simulink model "lab_1"  (R2025a)
settings: Solver=VariableStepAuto  StartTime=0.0  StopTime=20  RelTol=1e-3
model workspace (MAT data in the model file):
  K = Simulink.Parameter
  K.Value = 1.2
  K.Complexity = 'real'
  K.Dimensions = [1 1]
  K.DataType = 'auto'
  N = Simulink.Parameter
  N.Value = 100
  N.Complexity = 'real'
  N.Dimensions = [1 1]
  N.DataType = 'auto'
  T = Simulink.Parameter
  T.Value = 2.1
  T.Complexity = 'real'
  T.Dimensions = [1 1]
  T.DataType = 'auto'
  T_1 = Simulink.Parameter
  T_1.Value = 3.3
  T_1.Complexity = 'real'
  T_1.Dimensions = [1 1]
  T_1.DataType = 'auto'
  T_2 = Simulink.Parameter
  T_2.Value = 1.5
  T_2.Complexity = 'real'
  T_2.Dimensions = [1 1]
  T_2.DataType = 'auto'
  c_1 = Simulink.Parameter
  c_1.Value = 0.1
  c_1.Complexity = 'real'
  c_1.Dimensions = [1 1]
  c_1.DataType = 'auto'
  c_2 = Simulink.Parameter
  c_2.Value = 0.3
  c_2.Complexity = 'real'
  c_2.Dimensions = [1 1]
  c_2.DataType = 'auto'
  c_3 = Simulink.Parameter
  c_3.Value = 0.5
  c_3.Complexity = 'real'
  c_3.Dimensions = [1 1]
  c_3.DataType = 'auto'
settings Model: Creator=konstantin  LastModifiedBy=konstantin

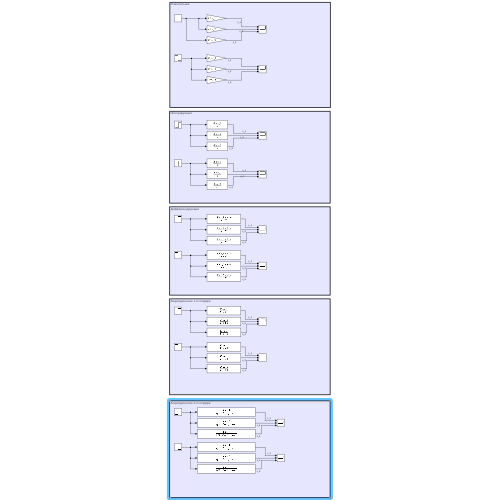
[thumbnail: Simulink's stored preview of the top-level diagram]
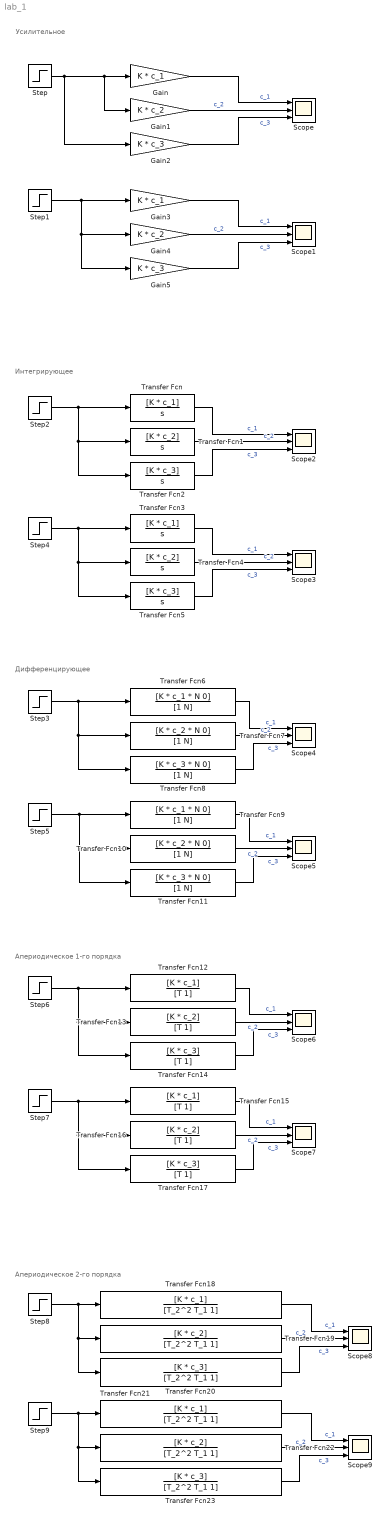
== system lab_1 ==
  note: Апериодическое 2-го порядка
  note: Апериодическое 1-го порядка
  note: Дифференцирующее
  note: Интегрирующее
  note: Усилительное
  Gain : Gain  Gain=K * c_1
  Gain1 : Gain  Gain=K * c_2
  Gain2 : Gain  Gain=K * c_3
  Gain3 : Gain  Gain=K * c_1
  Gain4 : Gain  Gain=K * c_2
  Gain5 : Gain  Gain=K * c_3
  Scope{,1..9} (10 alike) : Scope  NumInputPorts=3
      Scope settings: ActiveDisplayYMinimum=-1  ActiveDisplayYMaximum=1
      Scope1 settings: ActiveDisplayYMinimum=27.339308979558851  ActiveDisplayYMaximum=40.428766776937692
      Scope2 settings: ActiveDisplayYMinimum=-0.74999999999999978  ActiveDisplayYMaximum=6.75  DataLoggingVariableName=ScopeData2
      Scope3 settings: ActiveDisplayYMinimum=-0.74999999999999978  ActiveDisplayYMaximum=6.75  DataLoggingVariableName=ScopeData3
      Scope4 settings: ActiveDisplayYMinimum=-7.4999999999999982  ActiveDisplayYMaximum=67.5  DataLoggingVariableName=ScopeData4
      Scope5 settings: ActiveDisplayYMinimum=-7.4999999999999982  ActiveDisplayYMaximum=67.5  DataLoggingVariableName=ScopeData5
      Scope6 settings: ActiveDisplayYMinimum=-0.073967715995019639  ActiveDisplayYMaximum=0.66570944395517684  DataLoggingVariableName=ScopeData6
      Scope7 settings: ActiveDisplayYMinimum=-0.073967715995019639  ActiveDisplayYMaximum=0.66570944395517684  DataLoggingVariableName=ScopeData7
      Scope8 settings: ActiveDisplayYMinimum=-0.074962390858454561  ActiveDisplayYMaximum=0.67466151772609118  DataLoggingVariableName=ScopeData8
      Scope9 settings: ActiveDisplayYMinimum=-0.01724047204888899  ActiveDisplayYMaximum=0.15516424844000093  DataLoggingVariableName=ScopeData9
  Step : Step  Time=0  SampleTime=0
  Step{1,4..5,7,9} (5 alike) : Step  Time=0.01  Before=100  After=0  SampleTime=0
  Step2 : Step  Time=0  SampleTime=0
  Step3 : Step  SampleTime=0
  Step6 : Step  SampleTime=0
  Step8 : Step  SampleTime=0
  Transfer Fcn : TransferFcn  Numerator=[K * c_1]  Denominator=[1 0]
  Transfer Fcn1 : TransferFcn  Numerator=[K * c_2]  Denominator=[1 0]
  Transfer Fcn10 : TransferFcn  Numerator=[K * c_2 * N 0]  Denominator=[1 N]
  Transfer Fcn11 : TransferFcn  Numerator=[K * c_3 * N 0]  Denominator=[1 N]
  Transfer Fcn12 : TransferFcn  Numerator=[K * c_1]  Denominator=[T 1]
  Transfer Fcn13 : TransferFcn  Numerator=[K * c_2]  Denominator=[T 1]
  Transfer Fcn14 : TransferFcn  Numerator=[K * c_3]  Denominator=[T 1]
  Transfer Fcn15 : TransferFcn  Numerator=[K * c_1]  Denominator=[T 1]
  Transfer Fcn16 : TransferFcn  Numerator=[K * c_2]  Denominator=[T 1]
  Transfer Fcn17 : TransferFcn  Numerator=[K * c_3]  Denominator=[T 1]
  Transfer Fcn18 : TransferFcn  Numerator=[K * c_1]  Denominator=[T_2^2 T_1 1]
  Transfer Fcn19 : TransferFcn  Numerator=[K * c_2]  Denominator=[T_2^2 T_1 1]
  Transfer Fcn2 : TransferFcn  Numerator=[K * c_3]  Denominator=[1 0]
  Transfer Fcn20 : TransferFcn  Numerator=[K * c_3]  Denominator=[T_2^2 T_1 1]
  Transfer Fcn21 : TransferFcn  Numerator=[K * c_1]  Denominator=[T_2^2 T_1 1]
  Transfer Fcn22 : TransferFcn  Numerator=[K * c_2]  Denominator=[T_2^2 T_1 1]
  Transfer Fcn23 : TransferFcn  Numerator=[K * c_3]  Denominator=[T_2^2 T_1 1]
  Transfer Fcn3 : TransferFcn  Numerator=[K * c_1]  Denominator=[1 0]
  Transfer Fcn4 : TransferFcn  Numerator=[K * c_2]  Denominator=[1 0]
  Transfer Fcn5 : TransferFcn  Numerator=[K * c_3]  Denominator=[1 0]
  Transfer Fcn6 : TransferFcn  Numerator=[K * c_1 * N 0]  Denominator=[1 N]
  Transfer Fcn7 : TransferFcn  Numerator=[K * c_2 * N 0]  Denominator=[1 N]
  Transfer Fcn8 : TransferFcn  Numerator=[K * c_3 * N 0]  Denominator=[1 N]
  Transfer Fcn9 : TransferFcn  Numerator=[K * c_1 * N 0]  Denominator=[1 N]
  wires:
  Step/1 -> Gain1/1, Gain/1, Gain2/1
  Gain/1 -> Scope/1  "c_1"
  Gain1/1 -> Scope/2  "c_2"
  Gain2/1 -> Scope/3  "c_3"
  Step1/1 -> Gain5/1, Gain4/1, Gain3/1
  Gain4/1 -> Scope1/2  "c_2"
  Gain3/1 -> Scope1/1  "c_1"
  Gain5/1 -> Scope1/3  "c_3"
  Transfer Fcn1/1 -> Scope2/2  "c_2"
  Transfer Fcn/1 -> Scope2/1  "c_1"
  Step2/1 -> Transfer Fcn/1, Transfer Fcn2/1, Transfer Fcn1/1
  Transfer Fcn2/1 -> Scope2/3  "c_3"
  Transfer Fcn4/1 -> Scope3/2  "c_2"
  Step4/1 -> Transfer Fcn3/1, Transfer Fcn5/1, Transfer Fcn4/1
  Transfer Fcn5/1 -> Scope3/3  "c_3"
  Transfer Fcn3/1 -> Scope3/1  "c_1"
  Transfer Fcn7/1 -> Scope4/2  "c_2"
  Step3/1 -> Transfer Fcn6/1, Transfer Fcn8/1, Transfer Fcn7/1
  Transfer Fcn8/1 -> Scope4/3  "c_3"
  Transfer Fcn6/1 -> Scope4/1  "c_1"
  Transfer Fcn9/1 -> Scope5/1  "c_1"
  Transfer Fcn11/1 -> Scope5/3  "c_3"
  Transfer Fcn10/1 -> Scope5/2  "c_2"
  Step5/1 -> Transfer Fcn11/1, Transfer Fcn10/1, Transfer Fcn9/1
  Transfer Fcn12/1 -> Scope6/1  "c_1"
  Transfer Fcn14/1 -> Scope6/3  "c_3"
  Step6/1 -> Transfer Fcn12/1, Transfer Fcn14/1, Transfer Fcn13/1
  Transfer Fcn13/1 -> Scope6/2  "c_2"
  Transfer Fcn17/1 -> Scope7/3  "c_3"
  Transfer Fcn15/1 -> Scope7/1  "c_1"
  Transfer Fcn16/1 -> Scope7/2  "c_2"
  Step7/1 -> Transfer Fcn15/1, Transfer Fcn17/1, Transfer Fcn16/1
  Transfer Fcn20/1 -> Scope8/3  "c_3"
  Transfer Fcn18/1 -> Scope8/1  "c_1"
  Transfer Fcn19/1 -> Scope8/2  "c_2"
  Step8/1 -> Transfer Fcn18/1, Transfer Fcn19/1, Transfer Fcn20/1
  Step9/1 -> Transfer Fcn21/1, Transfer Fcn22/1, Transfer Fcn23/1
  Transfer Fcn23/1 -> Scope9/3  "c_3"
  Transfer Fcn22/1 -> Scope9/2  "c_2"
  Transfer Fcn21/1 -> Scope9/1  "c_1"
